simulink model "vloop_test"  (R2015b)
settings: Solver=ode15s  StartTime=0.0  StopTime=1.0  RelTol=1e-3
InitFcn:
  | G = 107.815;
libraries: simulink x1, roblocks x1
Description:
  | vloop parameters for
  | Puma560 shoulder joint
  | with link inertia
  | RVC1 p.205
settings Model: DisableUpgradeWarningsForVersion=R2014b  Creator=pic  LastModifiedBy=corkep
settings DataIOCC: SaveFormat=Array  SignalLoggingSaveFormat=ModelDataLogs  ReturnWorkspaceOutputs=on  TimeSaveName=t  OutputSaveName=y
settings OptimizationCC: ExpressionDepthLimit=2147483647
settings DebuggingCC: UnderspecifiedInitializationDetection=Classic  MergeDetectMultiDrivingBlocksExec=none  SolverPrmCheckMsg=warning  MultiTaskRateTransMsg=warning  FcnCallInpInsideContextMsg=UseLocalSettings  StateNameClashWarn=warning
settings HardwareCC: ProdBitPerPointer=32  ProdLargestAtomicFloat=None  ProdIntDivRoundTo=Undefined  ProdEndianess=Unspecified  ProdWordSize=32  ProdHWDeviceType=32-bit Generic
settings SFSimCC: SimCustomInitializer=|
  | if ~exist(tau_d)
  |    tau_d = 0
  | end
settings GRTTargetCC: GeneratePreprocessorConditionals=Disable all  CombineOutputUpdateFcns=off  GRTInterface=on
settings ConfigComp: CovModelRefEnable=Off  CovSFcnEnable=off

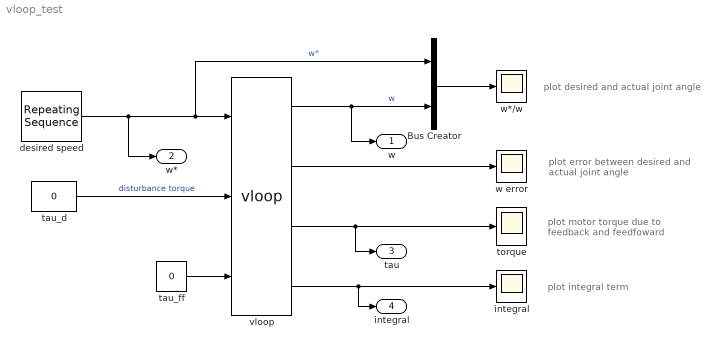
== system vloop_test ==
  note: plot integral term
  note: plot motor torque due
      | to feedback and feedfoward
  note: plot error between desired and
      | actual joint angle
  note: plot desired and actual joint angle
  Bus Creator : BusCreator  Inputs=2
  desired speed : simulink/Sources/Repeating Sequence  rep_seq_t=[0 1 3 4 6]/10  rep_seq_y=[0 0 50 50 0]
  "integral " : Scope
  tau_d : Constant  Value=0
  tau_ff : Constant  Value=0
  torque : Scope
  vloop : roblocks/Arm/vloop  J=580e-6  B=817e-6  Km=0.228  tau_max=0.9  Kv=0.6  Ki=0  T=0.001
  w error : Scope
  w*/w : Scope
  w : Outport
  w* : Outport  Port=2
  tau : Outport  Port=3
  integral : Outport  Port=4
  wires:
  desired speed/1 -> w*/1, Bus Creator/1, vloop/1  "w*"
  Bus Creator/1 -> w*/w/1
  vloop/1 -> Bus Creator/2, w/1  "w"
  vloop/2 -> w error/1
  vloop/3 -> tau/1, torque/1
  vloop/4 -> integral/1, "integral "/1
  tau_d/1 -> vloop/2  "disturbance torque"
  tau_ff/1 -> vloop/3
